simulink model "sampleModel1902_4_sub_sub"  (R2023a)
settings: Solver=VariableStepAuto  StartTime=0.0  StopTime=10.0  RelTol=1e-3
libraries: hdlsllib x4, simulink x1
settings Model: Creator=user1  LastModifiedBy=user1

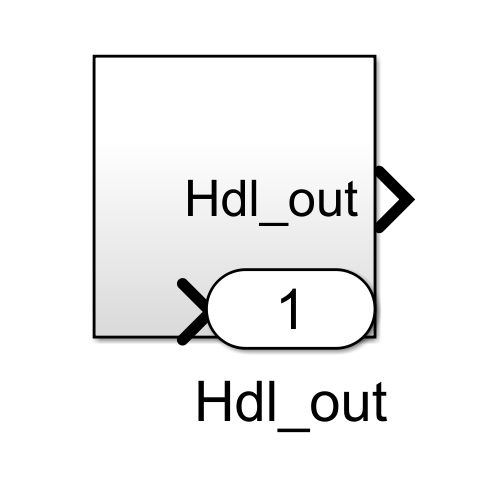
[thumbnail: Simulink's stored preview of the top-level diagram]
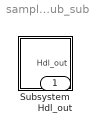
== system sampleModel1902_4_sub_sub ==
  Subsystem : Subsystem
  Hdl_out : Outport  OutDataTypeStr=uint8

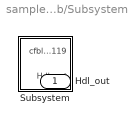
== system sampleModel1902_4_sub_sub/Subsystem ==
  Subsystem : Subsystem
  Hdl_out : Outport  OutDataTypeStr=uint8

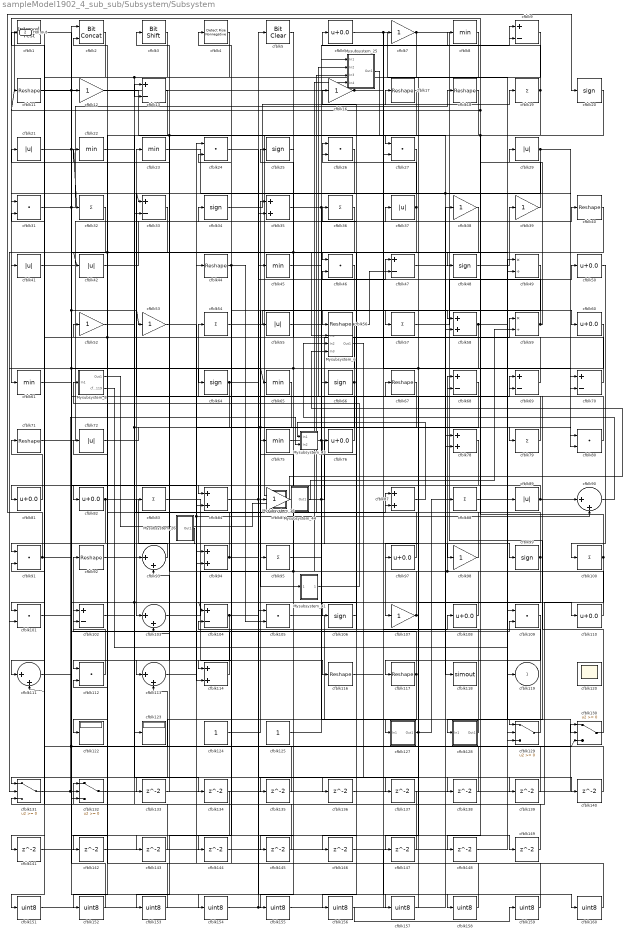
== system sampleModel1902_4_sub_sub/Subsystem/Subsystem ==
  Mysubsystem_16 : Subsystem  TreatAsAtomicUnit=on  RTWFcnName=Mysubsystem_16
      settings: RTWFcnNameOpts=User specified  RTWFileNameOpts=Use function name
  Mysubsystem_25 : Subsystem  TreatAsAtomicUnit=on  RTWFcnName=Mysubsystem_25
      settings: RTWFcnNameOpts=User specified  RTWFileNameOpts=Use function name
  Mysubsystem_26 : Subsystem  TreatAsAtomicUnit=on  RTWFcnName=Mysubsystem_26
      settings: RTWFcnNameOpts=User specified  RTWFileNameOpts=Use function name
  Mysubsystem_41 : Subsystem  TreatAsAtomicUnit=on  RTWFcnName=Mysubsystem_41
      settings: RTWFcnNameOpts=User specified  RTWFileNameOpts=Use function name
  Mysubsystem_43 : Subsystem  TreatAsAtomicUnit=on  RTWFcnName=Mysubsystem_43
      settings: RTWFcnNameOpts=User specified  RTWFileNameOpts=Use function name
  Mysubsystem_44 : Subsystem  TreatAsAtomicUnit=on  RTWFcnName=Mysubsystem_44
      settings: RTWFcnNameOpts=User specified  RTWFileNameOpts=Use function name
  Mysubsystem_6 : Subsystem  TreatAsAtomicUnit=on  RTWFcnName=Mysubsystem_6
      settings: RTWFcnNameOpts=User specified  RTWFileNameOpts=Use function name
  Mysubsystem_8 : Subsystem  TreatAsAtomicUnit=on  RTWFcnName=Mysubsystem_8
      settings: RTWFcnNameOpts=User specified  RTWFileNameOpts=Use function name
  cfblk1 : hdlsllib/Logic and Bit Operations/Interval Test  IntervalClosedRight=on  uplimit=0.5  IntervalClosedLeft=on  lowlimit=-0.5  OutDataTypeStr=uint8
  cfblk{19,32,36,54,57,79,83,88,95,100} (10 alike) : Sum  Inputs=+  OutDataTypeStr=uint8
  cfblk{24,26..27,31,46,80,91,101,105,109,112} (11 alike) : DotProduct  OutDataTypeStr=uint8
  cfblk{9,13,33,47,68..70,102,104} (9 alike) : Sum  Inputs=+-  OutDataTypeStr=uint8
  cfblk{90,93,103,111,113} (5 alike) : Sum  Inputs=|++  OutDataTypeStr=uint8
  cfblk{20,25,34,48,64,66,99,106} (8 alike) : Signum
  cfblk{7,12,16,38..39,52..53,85,98,107} (10 alike) : Gain  OutDataTypeStr=uint8
  cfblk{6,50,60,76,81..82,97,108,110} (9 alike) : Bias  Bias=0.0  SaturateOnIntegerOverflow=off
  cfblk{11,17..18,40,44,56,67,71,92,116..117} (11 alike) : Reshape
  cfblk{35,58,78,84,87,94,114} (7 alike) : Sum  OutDataTypeStr=uint8
  cfblk118 : ToWorkspace  VariableName=simout  SaveFormat=Timeseries  SampleTime=-1
  cfblk120 : Scope
      settings: Floating=on
  cfblk122 : Display
  cfblk123 : Display
  cfblk124 : Constant  OutDataTypeStr=uint8  SampleTime=-1
  cfblk125 : Constant  OutDataTypeStr=uint8  SampleTime=-1
  cfblk127 : Subsystem
      settings: LibrarySourceBlock=|
      | hdlsllib/Ports &
      | Subsystems/Subsystem
  cfblk128 : Subsystem
      settings: LibrarySourceBlock=|
      | hdlsllib/Ports &
      | Subsystems/Subsystem
  cfblk{129..132} (4 alike) : Switch  OutDataTypeStr=uint8  SaturateOnIntegerOverflow=off  InputSameDT=off
  cfblk{133..149} (17 alike) : Delay  SampleTime=1
  cfblk{151..160} (10 alike) : DataTypeConversion  OutDataTypeStr=uint8  SaturateOnIntegerOverflow=off  RndMeth=Floor
  cfblk2 : hdlsllib/Logic and Bit Operations/Bit Concat  numInputs=2
  cfblk{21,29,37,41..42,55,72,89} (8 alike) : Abs  OutDataTypeStr=uint8  SaturateOnIntegerOverflow=off
  cfblk{8,22..23,45,61,65,75} (7 alike) : MinMax  OutDataTypeStr=uint8
  cfblk3 : hdlsllib/Logic and Bit Operations/Bit Shift  mode=Shift Left Logical  N=0
  cfblk4 : hdlsllib/Logic and Bit Operations/Detect Rise Nonnegative  vinit=0  OutDataTypeStr=uint8
  cfblk49 : Product  Inputs=*/  OutDataTypeStr=uint8  RndMeth=Zero  SaturateOnIntegerOverflow=on
  cfblk5 : simulink/Logic and Bit Operations/Bit Clear  iBit=0
      settings: LibrarySourceBlock=|
      | hdlsllib/Logic and Bit
      | Operations/Bit Clear
  cfblk59 : Product  Inputs=*/  OutDataTypeStr=uint8  RndMeth=Zero  SaturateOnIntegerOverflow=on
  cfblk119 : Outport  OutDataTypeStr=uint8  VectorParamsAs1DForOutWhenUnconnected=off
  Hdl_out : Outport  Port=2  OutDataTypeStr=uint8
  wires:
  Mysubsystem_44/1(Out1) -> cfblk59/2
  cfblk87/1 -> Mysubsystem_43/1(In1)
  Mysubsystem_41/1(Out1) -> Mysubsystem_8/1(In1)
  Mysubsystem_26/1(Out1) -> cfblk99/1
  Mysubsystem_25/1(Out1) -> Mysubsystem_16/1(In1)
  cfblk97/1 -> Mysubsystem_25/3(In3)
  cfblk79/1 -> Mysubsystem_25/2(In2)
  Mysubsystem_16/1(Out1) -> Mysubsystem_6/3(In3)
  Mysubsystem_8/1(Out1) -> Mysubsystem_16/2(In2)
  Mysubsystem_8/2(cfblk119) -> cfblk119/1
  Mysubsystem_6/1(Out1) -> cfblk136/1
  cfblk90/1 -> Mysubsystem_6/2(In2)
  cfblk160/1 -> cfblk24/2
  cfblk146/1 -> cfblk160/1
  cfblk159/1 -> cfblk24/1
  cfblk156/1 -> cfblk159/1
  cfblk158/1 -> cfblk52/1
  cfblk24/1 -> cfblk158/1
  cfblk157/1 -> cfblk67/1
  cfblk67/1 -> cfblk156/1
  cfblk155/1 -> cfblk38/1
  cfblk5/1 -> cfblk155/1
  cfblk154/1 -> cfblk5/1
  cfblk111/1 -> cfblk154/1
  cfblk153/1 -> cfblk2/2
  cfblk134/1 -> cfblk153/1
  cfblk152/1 -> cfblk2/1
  cfblk13/1 -> cfblk152/1
  cfblk151/1 -> cfblk7/1, cfblk35/2
  cfblk149/1 -> cfblk104/2
  cfblk148/1 -> cfblk129/3
  cfblk147/1 -> cfblk13/1
  cfblk38/1 -> cfblk146/1
  cfblk145/1 -> cfblk1/1
  cfblk144/1 -> cfblk27/2
  cfblk143/1 -> cfblk112/2
  cfblk142/1 -> cfblk129/2
  cfblk141/1 -> cfblk49/1
  cfblk140/1 -> cfblk105/1
  cfblk139/1 -> cfblk91/2
  cfblk138/1 -> cfblk113/2
  cfblk137/1 -> cfblk131/3
  cfblk18/1 -> cfblk137/1
  cfblk136/1 -> cfblk130/1
  cfblk135/1 -> cfblk93/2
  cfblk133/1 -> cfblk103/2
  cfblk2/1 -> cfblk151/1
  cfblk35/1 -> cfblk19/1, cfblk58/1
  cfblk93/1 -> cfblk91/1
  cfblk130/1 -> cfblk69/1
  cfblk102/1 -> cfblk87/2
  cfblk26/1 -> cfblk111/1
  cfblk64/1 -> cfblk94/2, cfblk138/1
  cfblk132/1 -> cfblk78/1
  cfblk37/1 -> Mysubsystem_6/1(In1), cfblk26/2
  cfblk47/1 -> cfblk60/1
  cfblk52/1 -> cfblk123/1, cfblk104/1
  cfblk9/1 -> cfblk41/1
  cfblk127/1(Out1) -> cfblk87/1, cfblk88/1
  cfblk56/1 -> cfblk101/2, cfblk135/1, cfblk47/2
  cfblk45/1 -> cfblk129/1
  cfblk1/1 -> cfblk111/2, cfblk157/1
  cfblk103/1 -> cfblk45/1
  cfblk4/1 -> cfblk132/2, cfblk13/2
  cfblk95/1 -> cfblk9/1
  cfblk101/1 -> cfblk68/2
  cfblk50/1 -> cfblk100/1
  cfblk117/1 -> cfblk102/2, cfblk133/1
  cfblk125/1 -> cfblk66/1
  cfblk53/1 -> cfblk94/1
  cfblk16/1 -> cfblk70/2, Hdl_out/1
  cfblk17/1 -> cfblk113/1, cfblk33/2
  cfblk61/1 -> cfblk110/1
  cfblk25/1 -> cfblk85/1
  cfblk89/1 -> cfblk84/1, cfblk90/1
  cfblk104/1 -> cfblk112/1, cfblk69/2
  cfblk114/1 -> cfblk102/1
  cfblk84/1 -> cfblk47/1, cfblk140/1
  cfblk88/1 -> cfblk89/1
  cfblk66/1 -> cfblk25/1, cfblk114/2
  cfblk92/1 -> cfblk93/1
  cfblk72/1 -> cfblk79/1
  cfblk22/1 -> cfblk80/2, cfblk134/1
  cfblk12/1 -> cfblk118/1
  cfblk131/1 -> Mysubsystem_43/2(In2), cfblk109/2, cfblk130/3
  cfblk3/1 -> cfblk101/1
  cfblk68/1 -> cfblk106/1
  cfblk128/1(Out1) -> cfblk76/1
  cfblk83/1 -> cfblk116/1
  cfblk81/1 -> cfblk71/1
  cfblk78/1 -> cfblk81/1
  cfblk107/1 -> cfblk36/1, cfblk147/1
  cfblk94/1 -> cfblk72/1, cfblk139/1
  cfblk36/1 -> cfblk42/1, cfblk145/1
  cfblk57/1 -> cfblk50/1
  cfblk39/1 -> cfblk6/1, cfblk11/1
  cfblk98/1 -> cfblk83/1
  cfblk32/1 -> cfblk131/2
  cfblk110/1 -> cfblk21/1, cfblk75/1
  cfblk69/1 -> cfblk22/1, cfblk31/2
  cfblk29/1 -> cfblk33/1, cfblk58/2, cfblk80/1
  cfblk106/1 -> cfblk46/2
  cfblk58/1 -> cfblk122/1, cfblk130/2
  cfblk85/1 -> cfblk59/1, cfblk9/2
  cfblk44/1 -> cfblk64/1, cfblk105/2
  cfblk20/1 -> cfblk55/1
  cfblk70/1 -> cfblk3/1
  cfblk8/1 -> cfblk27/1
  cfblk42/1 -> cfblk37/1
  cfblk55/1 -> cfblk57/1
  cfblk82/1 -> cfblk98/1, cfblk132/3
  cfblk21/1 -> cfblk84/2, cfblk65/1, cfblk53/1, cfblk32/1
  cfblk33/1 -> cfblk141/1, cfblk142/1
  cfblk75/1 -> Mysubsystem_25/1(In1), cfblk107/1
  cfblk49/1 -> cfblk95/1
  cfblk54/1 -> cfblk56/1
  cfblk6/1 -> cfblk109/1, cfblk49/2
  cfblk27/1 -> cfblk103/1
  cfblk48/1 -> cfblk39/1
  cfblk80/1 -> cfblk54/1
  cfblk100/1 -> cfblk132/1, cfblk8/1
  cfblk91/1 -> cfblk20/1, cfblk149/1
  cfblk129/1 -> cfblk4/1
  cfblk108/1 -> Mysubsystem_25/4(In4), cfblk68/1
  cfblk11/1 -> cfblk12/1, cfblk143/1
  cfblk31/1 -> cfblk18/1, cfblk48/1
  cfblk76/1 -> cfblk23/1
  cfblk116/1 -> cfblk108/1
  cfblk46/1 -> cfblk114/1
  cfblk113/1 -> cfblk44/1, cfblk90/2
  cfblk23/1 -> cfblk70/1
  cfblk65/1 -> Mysubsystem_41/1(In1), cfblk144/1
  cfblk59/1 -> cfblk26/1, cfblk29/1
  cfblk60/1 -> cfblk82/1, cfblk97/1
  cfblk109/1 -> cfblk117/1
  cfblk19/1 -> cfblk78/2, cfblk148/1, cfblk61/1
  cfblk99/1 -> cfblk131/1, cfblk16/1
  cfblk124/1 -> cfblk35/1
  cfblk71/1 -> cfblk40/1
  cfblk40/1 -> cfblk46/1
  cfblk105/1 -> cfblk127/1(In1)
  cfblk7/1 -> cfblk128/1(In1), cfblk31/1
  cfblk41/1 -> cfblk34/1
  cfblk34/1 -> cfblk17/1
  cfblk112/1 -> cfblk92/1

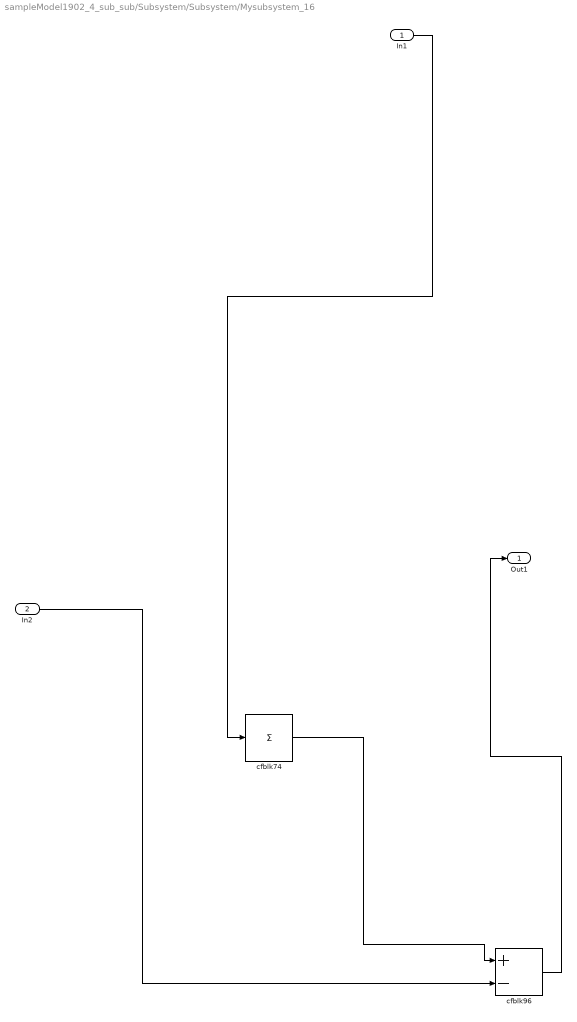
== system sampleModel1902_4_sub_sub/Subsystem/Subsystem/Mysubsystem_16 ==
  In1 : Inport
  In2 : Inport  Port=2
  cfblk74 : Sum  Inputs=+
  cfblk96 : Sum  Inputs=+-
  Out1 : Outport
  wires:
  cfblk74/1 -> cfblk96/1
  cfblk96/1 -> Out1/1
  In1/1 -> cfblk74/1
  In2/1 -> cfblk96/2

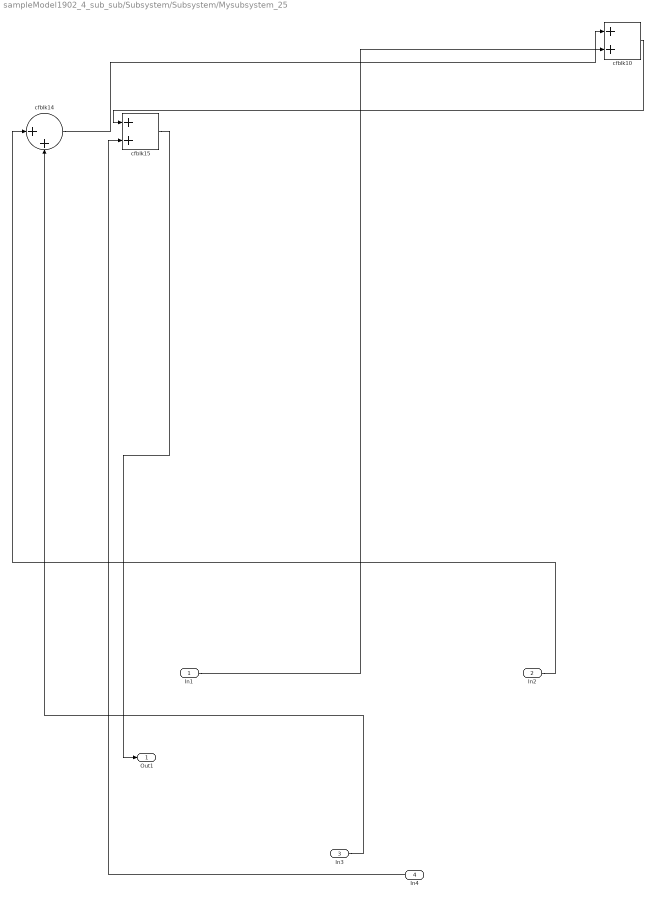
== system sampleModel1902_4_sub_sub/Subsystem/Subsystem/Mysubsystem_25 ==
  In1 : Inport
  In2 : Inport  Port=2
  In3 : Inport  Port=3
  In4 : Inport  Port=4
  cfblk10 : Sum
  cfblk14 : Sum  Inputs=|++
  cfblk15 : Sum
  Out1 : Outport
  wires:
  cfblk10/1 -> cfblk15/1
  cfblk14/1 -> cfblk10/1
  In2/1 -> cfblk14/1
  cfblk15/1 -> Out1/1
  In3/1 -> cfblk14/2
  In4/1 -> cfblk15/2
  In1/1 -> cfblk10/2

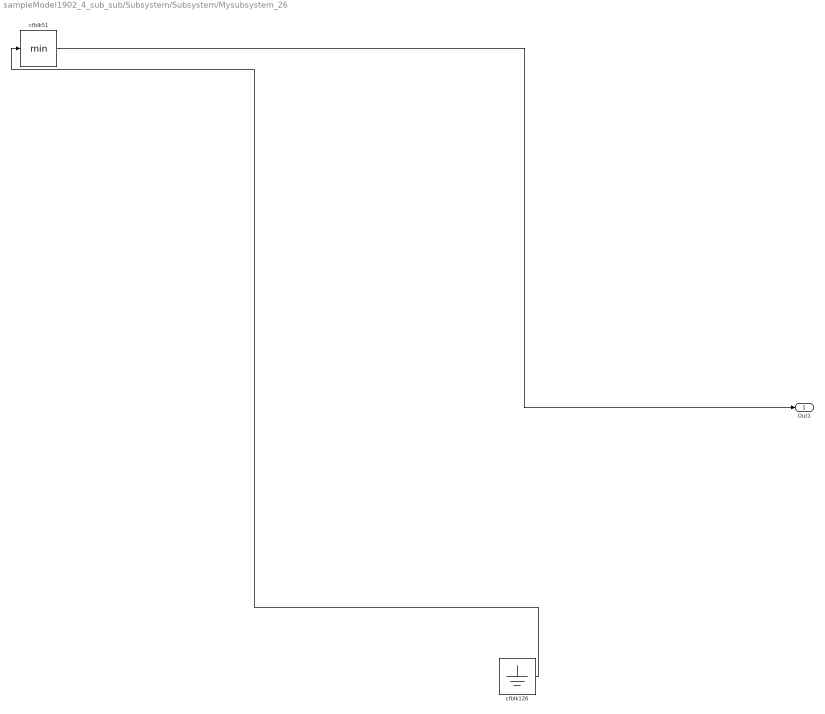
== system sampleModel1902_4_sub_sub/Subsystem/Subsystem/Mysubsystem_26 ==
  cfblk126 : Ground
  cfblk51 : MinMax
  Out1 : Outport
  wires:
  cfblk126/1 -> cfblk51/1
  cfblk51/1 -> Out1/1

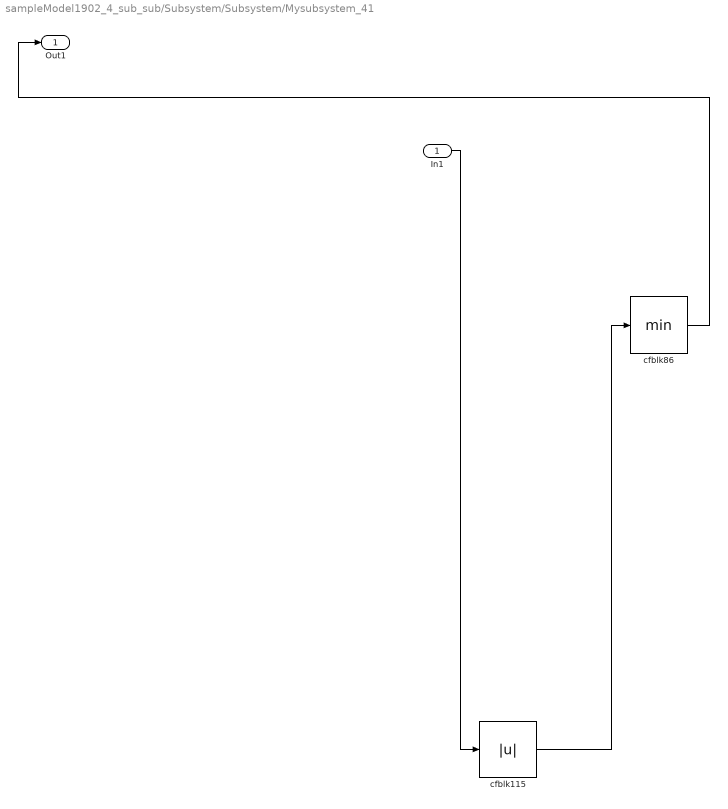
== system sampleModel1902_4_sub_sub/Subsystem/Subsystem/Mysubsystem_41 ==
  In1 : Inport
  cfblk115 : Abs  SaturateOnIntegerOverflow=off
  cfblk86 : MinMax
  Out1 : Outport
  wires:
  cfblk86/1 -> Out1/1
  cfblk115/1 -> cfblk86/1
  In1/1 -> cfblk115/1

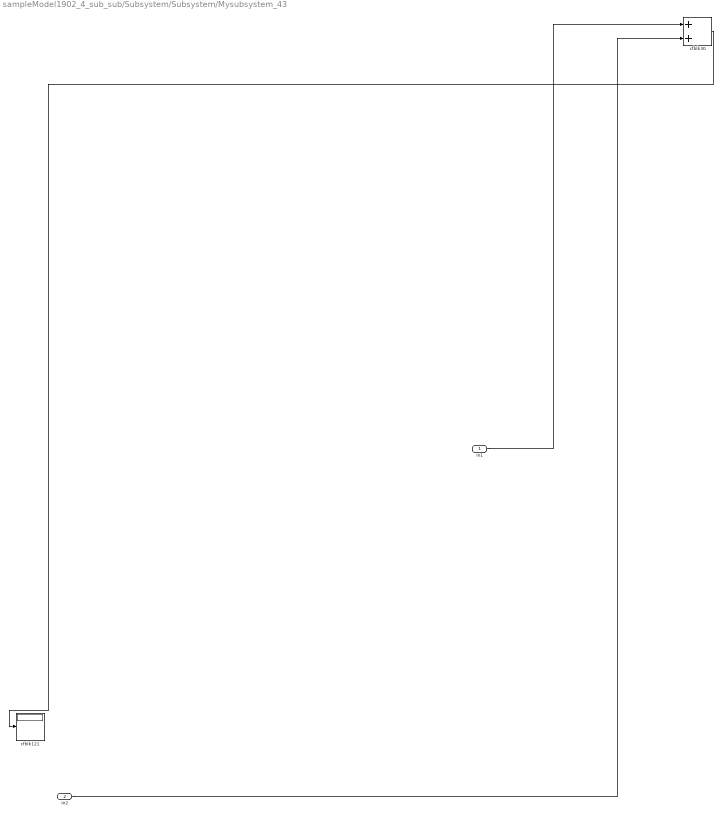
== system sampleModel1902_4_sub_sub/Subsystem/Subsystem/Mysubsystem_43 ==
  In1 : Inport
  In2 : Inport  Port=2
  cfblk121 : Display
  cfblk30 : Sum
  wires:
  cfblk30/1 -> cfblk121/1
  In1/1 -> cfblk30/1
  In2/1 -> cfblk30/2

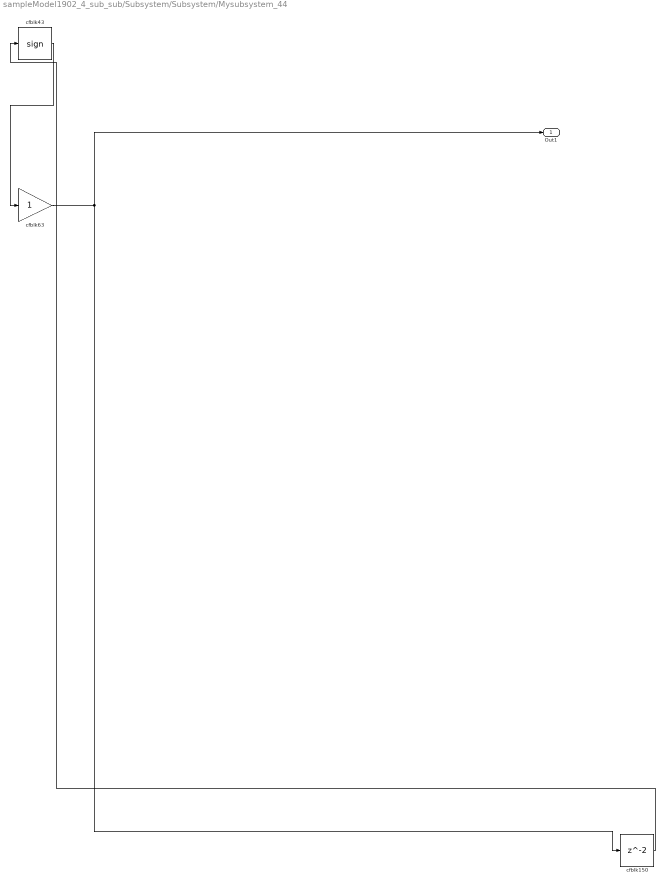
== system sampleModel1902_4_sub_sub/Subsystem/Subsystem/Mysubsystem_44 ==
  cfblk150 : Delay  SampleTime=1
  cfblk43 : Signum
  cfblk63 : Gain
  Out1 : Outport
  wires:
  cfblk150/1 -> cfblk43/1
  cfblk63/1 -> Out1/1, cfblk150/1
  cfblk43/1 -> cfblk63/1

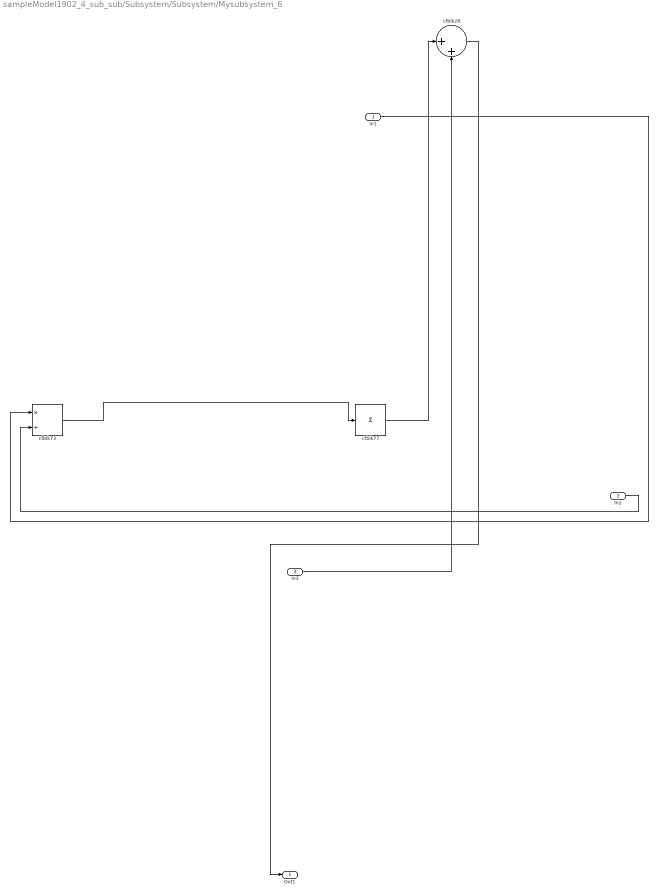
== system sampleModel1902_4_sub_sub/Subsystem/Subsystem/Mysubsystem_6 ==
  In1 : Inport
  In2 : Inport  Port=2
  In3 : Inport  Port=3
  cfblk28 : Sum  Inputs=|++
  cfblk73 : Product  Inputs=*/  RndMeth=Zero  SaturateOnIntegerOverflow=on
  cfblk77 : Sum  Inputs=+
  Out1 : Outport
  wires:
  In3/1 -> cfblk28/2
  cfblk73/1 -> cfblk77/1
  cfblk77/1 -> cfblk28/1
  cfblk28/1 -> Out1/1
  In2/1 -> cfblk73/2
  In1/1 -> cfblk73/1

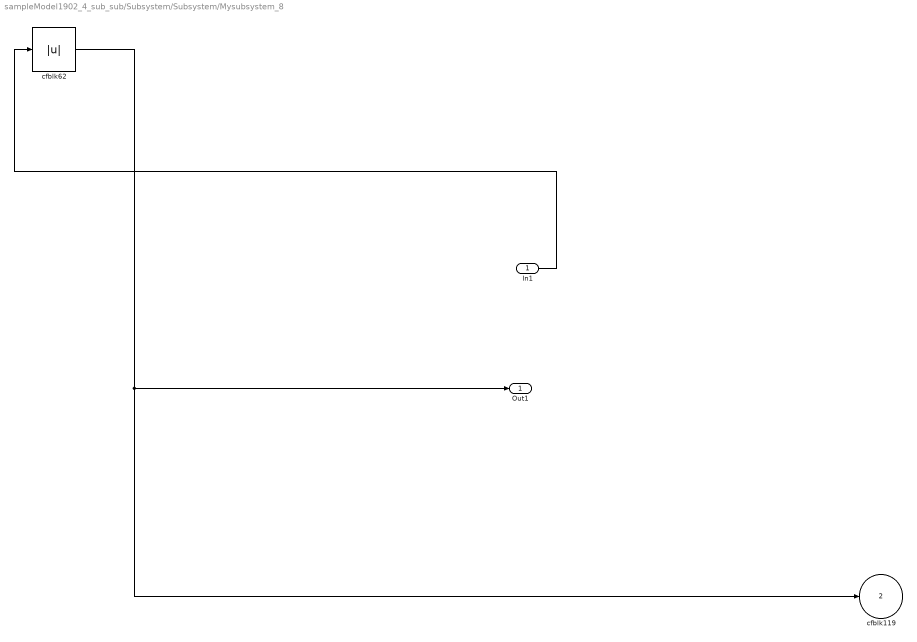
== system sampleModel1902_4_sub_sub/Subsystem/Subsystem/Mysubsystem_8 ==
  In1 : Inport
  cfblk62 : Abs  SaturateOnIntegerOverflow=off
  Out1 : Outport
  cfblk119 : Outport  Port=2  VectorParamsAs1DForOutWhenUnconnected=off
  wires:
  cfblk62/1 -> cfblk119/1, Out1/1
  In1/1 -> cfblk62/1

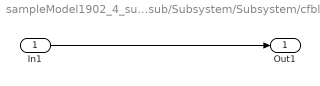
== system sampleModel1902_4_sub_sub/Subsystem/Subsystem/cfblk127 ==
  In1 : Inport
  Out1 : Outport
  wires:
  In1/1 -> Out1/1

== system sampleModel1902_4_sub_sub/Subsystem/Subsystem/cfblk128 ==
  In1 : Inport
  Out1 : Outport
  wires:
  In1/1 -> Out1/1
